simulink model "discrete_time_model"  (R2024b)
settings: Solver=FixedStepAuto  StartTime=0.0  StopTime=2  FixedStep=0.1  RelTol=1e-3
undefined symbols (not defined in the file or in its folder): K_LQR
settings Model: Creator=root  LastModifiedBy=root

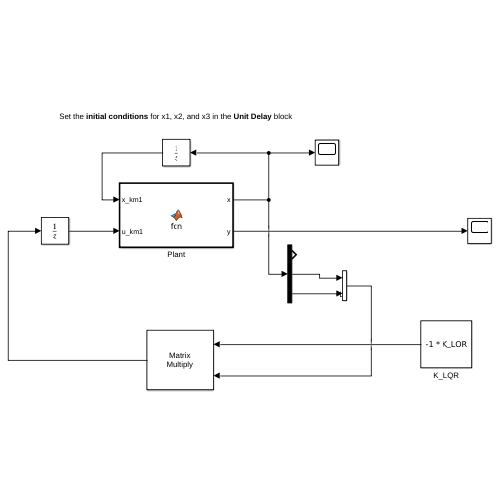
[thumbnail: Simulink's stored preview of the top-level diagram]
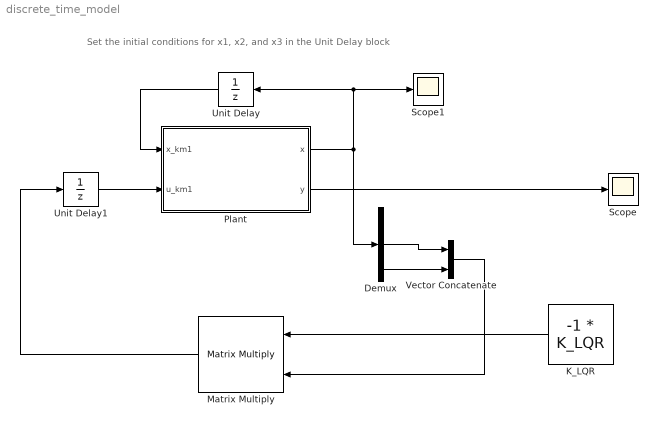
== system discrete_time_model ==
  note: Set the initial conditions for x1, x2, and x3 in the Unit Delay block
  Demux : Demux  Outputs=3
  K_LQR : Constant  Value=-1 * K_LQR  VectorParams1D=off
  Matrix Multiply : Product  Multiplication=Matrix(*)
  Plant : MATLAB Function  TreatAsAtomicUnit=on
  Scope : Scope
  Scope1 : Scope
  Unit Delay : UnitDelay  InitialCondition=[5; 5; 0]  SampleTime=-1  HasFrameUpgradeWarning=on
  Unit Delay1 : UnitDelay  SampleTime=-1  HasFrameUpgradeWarning=on
  Vector Concatenate : Concatenate  Mode=Multidimensional array
  wires:
  Plant/1(x) -> Demux/1, Scope1/1, Unit Delay/1
  Plant/2(y) -> Scope/1
  Unit Delay/1 -> Plant/1(x_km1)
  K_LQR/1 -> Matrix Multiply/1
  Matrix Multiply/1 -> Unit Delay1/1
  Demux/2 -> Vector Concatenate/1
  Demux/3 -> Vector Concatenate/2
  Vector Concatenate/1 -> Matrix Multiply/2
  Unit Delay1/1 -> Plant/2(u_km1)

== matlab function discrete_time_model/Plant ==
  data: x_km1 input; u_km1 input; x output; y output
% km1 = k minus 1
function [x, y] = fcn( x_km1, u_km1)

x1_km1 = x_km1(1);
x2_km1 = x_km1(2);
x3_km1 = x_km1(3);

x1 = x1_km1;
x2 = x2_km1 + x3_km1;
x3 = x3_km1 + u_km1;

y1 = x1*cos(deg2rad(x2));
y2 = x1_km1*cos(deg2rad(x2_km1));

x = [x1; x2; x3];
y = [y1; y2];
